simulink model "project_mass"  (R2024b)
settings: Solver=VariableStepAuto  StartTime=0.0  StopTime=sim_time  MaxStep=0.01  RelTol=1e-3
values from neighbouring files (symbols this model uses):
  b = 10    [PID_Tune.m]    (also in Pid_Basics.m; electric_M.m = 3.5077e-06; pid_script.m = 20; practice.m = 40)
  F = 2    [project_1.m]    (also in project_m1.m = 1; project_mass_m.m = 1)
  k = 20    [PID_Tune.m]    (also in Pid_Basics.m; project_m1.m; project_mass_m.m)
settings Model: Creator=vishwanth  LastModifiedBy=vishwanth

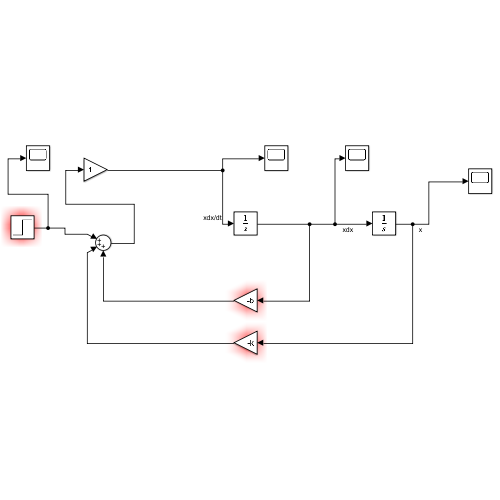
[thumbnail: Simulink's stored preview of the top-level diagram]
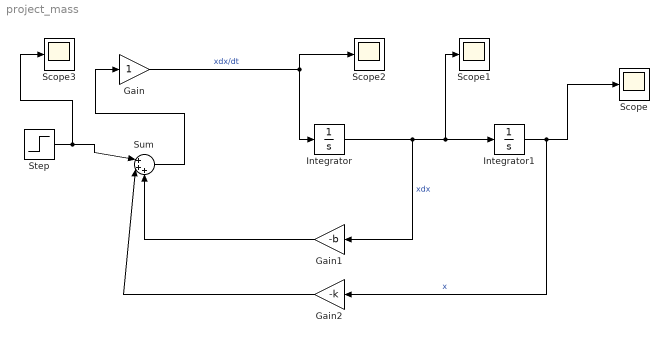
== system project_mass ==
  Gain : Gain
  Gain1 : Gain  Gain=-b
  Gain2 : Gain  Gain=-k
  Integrator : Integrator
  Integrator1 : Integrator
  Scope{,1..3} (4 alike) : Scope
  Step : Step  After=F  SampleTime=0
  Sum : Sum  Inputs=|+++
  wires:
  Integrator/1 -> Gain1/1, Scope1/1, Integrator1/1  "xdx"
  Gain/1 -> Scope2/1, Integrator/1  "xdx/dt"
  Integrator1/1 -> Gain2/1, Scope/1  "x"
  Gain1/1 -> Sum/3
  Gain2/1 -> Sum/2
  Step/1 -> Scope3/1, Sum/1
  Sum/1 -> Gain/1
